simulink library "three_phase_voltage_emulator"  (R2025b)
settings: Solver=VariableStepAuto  StartTime=0.0  StopTime=10.0  RelTol=1e-3
libraries: cstblocks x4
settings Model: Creator=dbagn  LastModifiedBy=dbagn

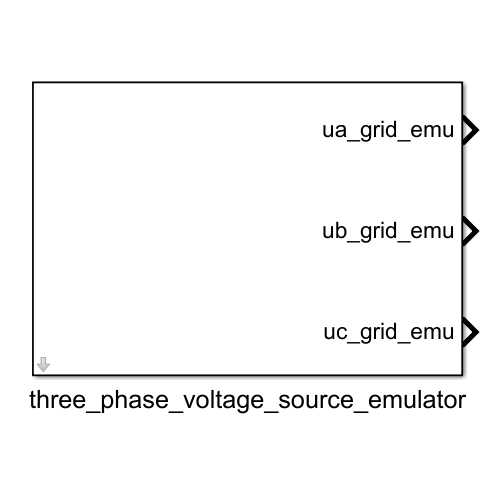
[thumbnail: Simulink's stored preview of the top-level diagram]
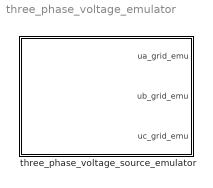
== system three_phase_voltage_emulator ==
  three_phase_voltage_source_emulator : Subsystem  mask{omega_grid_emulator_nom=2*pi*50, ugrid_nom=690, vp_xi_pu=1, vp_eta_pu=0, vn_xi_pu=0, vn_eta_pu=0, fcut_lvrt=50, LVRT_flt_ss=1, ugrid_phase=0}
      mask prompts: omega_grid_emulator_nom "Nominal Pulsation [rad/s]"; ugrid_nom "Nominal Voltage [V]"; vp_xi_pu "vp_xi_pu [pu]"; vp_eta_pu "vp_eta_pu [pu]"; vn_xi_pu "vn_xi_pu [pu]"; vn_eta_pu "vn_eta_pu [pu]"; fcut_lvrt "LVRT LPF [Hz]"

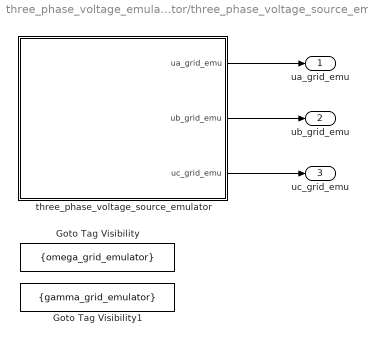
== system three_phase_voltage_emulator/three_phase_voltage_source_emulator ==
  Goto Tag Visibility : GotoTagVisibility  GotoTag=omega_grid_emulator
  Goto Tag Visibility1 : GotoTagVisibility  GotoTag=gamma_grid_emulator
  three_phase_voltage_source_emulator : Subsystem
  ua_grid_emu : Outport  VectorParamsAs1DForOutWhenUnconnected=off
  ub_grid_emu : Outport  Port=2  VectorParamsAs1DForOutWhenUnconnected=off
  uc_grid_emu : Outport  Port=3  VectorParamsAs1DForOutWhenUnconnected=off
  wires:
  three_phase_voltage_source_emulator/1(ua_grid_emu) -> ua_grid_emu/1
  three_phase_voltage_source_emulator/2(ub_grid_emu) -> ub_grid_emu/1
  three_phase_voltage_source_emulator/3(uc_grid_emu) -> uc_grid_emu/1

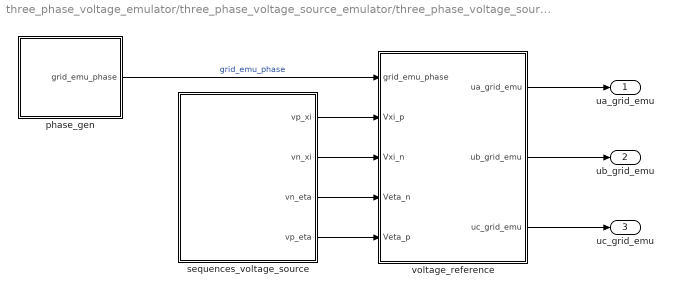
== system three_phase_voltage_emulator/three_phase_voltage_source_emulator/three_phase_voltage_source_emulator ==
  phase_gen : Subsystem
  sequences_voltage_source : Subsystem
  voltage_reference : Subsystem
  ua_grid_emu : Outport  VectorParamsAs1DForOutWhenUnconnected=off
  ub_grid_emu : Outport  Port=2  VectorParamsAs1DForOutWhenUnconnected=off
  uc_grid_emu : Outport  Port=3  VectorParamsAs1DForOutWhenUnconnected=off
  wires:
  phase_gen/1(grid_emu_phase) -> voltage_reference/1(grid_emu_phase)  "grid_emu_phase"
  sequences_voltage_source/2(vn_xi) -> voltage_reference/3(Vxi_n)
  sequences_voltage_source/1(vp_xi) -> voltage_reference/2(Vxi_p)
  sequences_voltage_source/3(vn_eta) -> voltage_reference/4(Veta_n)
  voltage_reference/3(uc_grid_emu) -> uc_grid_emu/1
  voltage_reference/1(ua_grid_emu) -> ua_grid_emu/1
  voltage_reference/2(ub_grid_emu) -> ub_grid_emu/1
  sequences_voltage_source/4(vp_eta) -> voltage_reference/5(Veta_p)

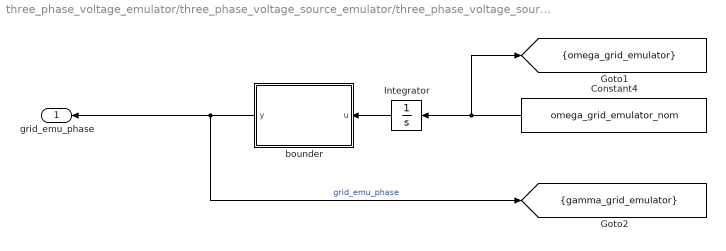
== system three_phase_voltage_emulator/three_phase_voltage_source_emulator/three_phase_voltage_source_emulator/phase_gen ==
  Constant4 : Constant  Value=omega_grid_emulator_nom
  Integrator : Integrator
  bounder : MATLAB Function  TreatAsAtomicUnit=on
  grid_emu_phase : Outport  VectorParamsAs1DForOutWhenUnconnected=off
  tag scope: gamma_grid_emulator=scoped, omega_grid_emulator=scoped
  wires:
  bounder/1(y) -> [gamma_grid_emulator], grid_emu_phase/1  "grid_emu_phase"
  Constant4/1 -> [omega_grid_emulator], Integrator/1
  Integrator/1 -> bounder/1(u)

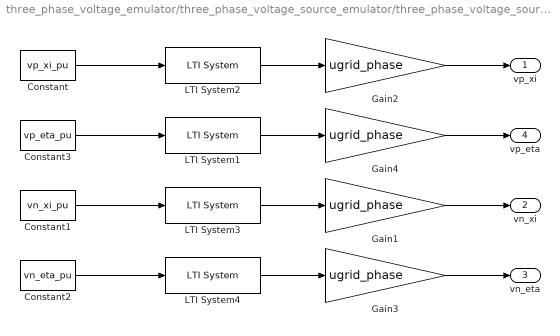
== system three_phase_voltage_emulator/three_phase_voltage_source_emulator/three_phase_voltage_source_emulator/sequences_voltage_source ==
  Constant : Constant  Value=vp_xi_pu
  Constant1 : Constant  Value=vn_xi_pu
  Constant2 : Constant  Value=vn_eta_pu
  Constant3 : Constant  Value=vp_eta_pu
  Gain{1..4} (4 alike) : Gain  Gain=ugrid_phase
  LTI System{1..4} (4 alike) : cstblocks/LTI System  sys=LVRT_flt_ss  IC=[0]  PadeOrder=0
  vp_xi : Outport  VectorParamsAs1DForOutWhenUnconnected=off
  vn_xi : Outport  Port=2  VectorParamsAs1DForOutWhenUnconnected=off
  vn_eta : Outport  Port=3  VectorParamsAs1DForOutWhenUnconnected=off
  vp_eta : Outport  Port=4  VectorParamsAs1DForOutWhenUnconnected=off
  wires:
  LTI System2/1 -> Gain2/1
  LTI System3/1 -> Gain1/1
  LTI System4/1 -> Gain3/1
  Gain2/1 -> vp_xi/1
  Gain1/1 -> vn_xi/1
  Gain3/1 -> vn_eta/1
  Constant2/1 -> LTI System4/1
  Constant/1 -> LTI System2/1
  Constant1/1 -> LTI System3/1
  Constant3/1 -> LTI System1/1
  Gain4/1 -> vp_eta/1
  LTI System1/1 -> Gain4/1

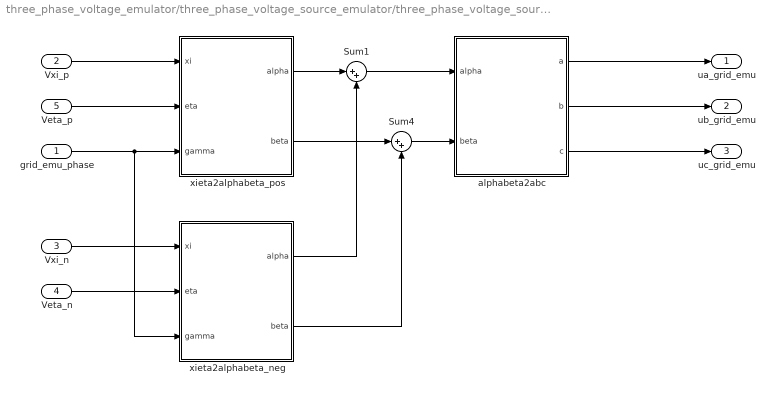
== system three_phase_voltage_emulator/three_phase_voltage_source_emulator/three_phase_voltage_source_emulator/voltage_reference ==
  grid_emu_phase : Inport
  Vxi_p : Inport  Port=2
  Vxi_n : Inport  Port=3
  Veta_n : Inport  Port=4
  Veta_p : Inport  Port=5
  Sum1 : Sum  Inputs=|++
  Sum4 : Sum  Inputs=|++
  alphabeta2abc : MATLAB Function  TreatAsAtomicUnit=on
  xieta2alphabeta_neg : MATLAB Function  TreatAsAtomicUnit=on
  xieta2alphabeta_pos : MATLAB Function  TreatAsAtomicUnit=on
  ua_grid_emu : Outport  VectorParamsAs1DForOutWhenUnconnected=off
  ub_grid_emu : Outport  Port=2  VectorParamsAs1DForOutWhenUnconnected=off
  uc_grid_emu : Outport  Port=3  VectorParamsAs1DForOutWhenUnconnected=off
  wires:
  xieta2alphabeta_pos/1(alpha) -> Sum1/1
  Sum1/1 -> alphabeta2abc/1(alpha)
  xieta2alphabeta_pos/2(beta) -> Sum4/1
  Sum4/1 -> alphabeta2abc/2(beta)
  xieta2alphabeta_neg/1(alpha) -> Sum1/2
  xieta2alphabeta_neg/2(beta) -> Sum4/2
  grid_emu_phase/1 -> xieta2alphabeta_neg/3(gamma), xieta2alphabeta_pos/3(gamma)
  Vxi_p/1 -> xieta2alphabeta_pos/1(xi)
  Veta_p/1 -> xieta2alphabeta_pos/2(eta)
  Vxi_n/1 -> xieta2alphabeta_neg/1(xi)
  Veta_n/1 -> xieta2alphabeta_neg/2(eta)
  alphabeta2abc/2(b) -> ub_grid_emu/1
  alphabeta2abc/3(c) -> uc_grid_emu/1
  alphabeta2abc/1(a) -> ua_grid_emu/1

== matlab function three_phase_voltage_emulator/three_phase_voltage_source_emulator/three_phase_voltage_source_emulator/voltage_reference/alphabeta2abc ==
  data: alpha input; a output; beta input; b output; c output
function [a,b,c] = alphabeta2abc(alpha,beta)

    a  =  alpha;
    b  =  -0.5*alpha + sqrt(3)/2*beta;
    c  =  -0.5*alpha - sqrt(3)/2*beta;
end

== matlab function three_phase_voltage_emulator/three_phase_voltage_source_emulator/three_phase_voltage_source_emulator/voltage_reference/xieta2alphabeta_neg ==
  data: xi input; alpha output; eta input; gamma input; beta output
function [alpha,beta] = xieta2alphabeta_neg(xi,eta,gamma)

    alpha  =  xi*cos(gamma) + eta*sin(gamma);
    beta = -xi*sin(gamma) + eta*cos(gamma);

end

== matlab function three_phase_voltage_emulator/three_phase_voltage_source_emulator/three_phase_voltage_source_emulator/voltage_reference/xieta2alphabeta_pos ==
  data: xi input; alpha output; eta input; gamma input; beta output
function [alpha,beta] = xieta2alphabeta_pos(xi,eta,gamma)

    alpha  =  xi*cos(gamma) - eta*sin(gamma);
    beta = xi*sin(gamma) + eta*cos(gamma);

end

== matlab function three_phase_voltage_emulator/three_phase_voltage_source_emulator/three_phase_voltage_source_emulator/phase_gen/bounder ==
  data: u input; y output
function y = bounder(u)    
    y = -pi + mod(u+3*pi,2*pi);
end
